simulink model "Seat_PC_Model"  (R2020a)
settings: Solver=FixedStepDiscrete  StartTime=0.0  StopTime=30  FixedStep=1  RelTol=1e-3
undefined symbols (not defined in the file or in its folder): Seat_PC_System
libraries: simulink x2
settings Model: Creator=A  LastModifiedBy=A

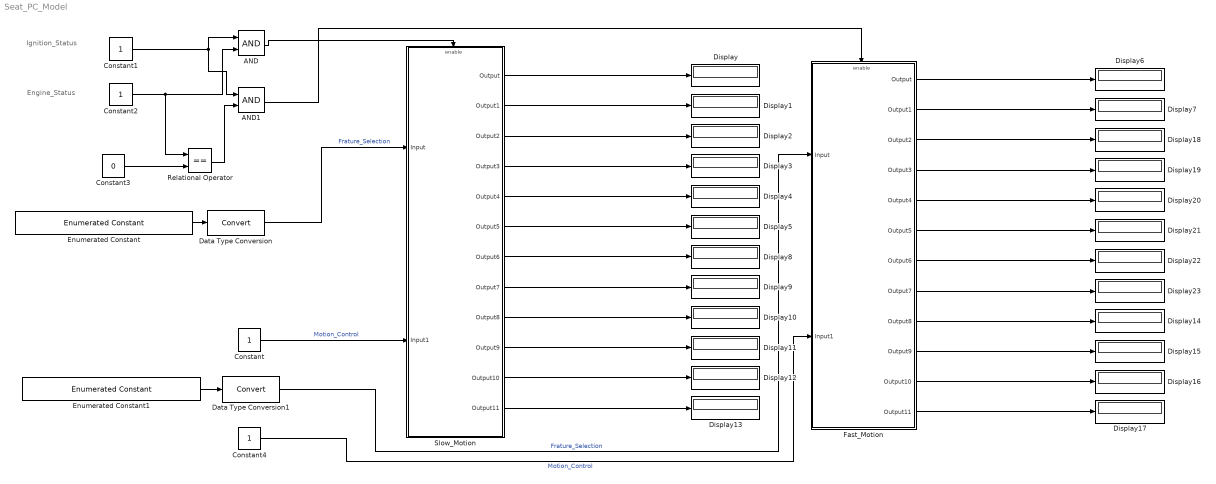
== system Seat_PC_Model ==
  note: Engine_Status
  note: Ignition_Status
  AND : Logic  AllPortsSameDT=off  OutDataTypeStr=boolean
  AND1 : Logic  AllPortsSameDT=off  OutDataTypeStr=boolean
  Constant{,1..2,4} (4 alike) : Constant  OutDataTypeStr=boolean
  Constant3 : Constant  Value=0  OutDataTypeStr=boolean
  Data Type Conversion : DataTypeConversion
  Data Type Conversion1 : DataTypeConversion
  Display{,1..23} (24 alike) : Display
  Enumerated Constant : simulink/Sources/Enumerated Constant  OutDataTypeStr=Enum:Seat_PC_System  Value=Seat_PC_System.SeatBack_FrontTilt_RearTilt_Recline_M  SampleTime=inf
  Enumerated Constant1 : simulink/Sources/Enumerated Constant  OutDataTypeStr=Enum:Seat_PC_System  Value=Seat_PC_System.Headrest_Upward_Downward_M  SampleTime=inf
  Fast_Motion : Subsystem
  Relational Operator : RelationalOperator  Operator===  OutDataTypeStr=boolean  RndMeth=Simplest
  Slow_Motion : Subsystem
  wires:
  AND/1 -> Slow_Motion/Enable
  AND1/1 -> Fast_Motion/Enable
  Constant1/1 -> AND1/1, AND/1
  Constant2/1 -> Relational Operator/1, AND/2
  Constant3/1 -> Relational Operator/2
  Relational Operator/1 -> AND1/2
  Slow_Motion/1(Output) -> Display/1
  Slow_Motion/2(Output1) -> Display1/1
  Slow_Motion/3(Output2) -> Display2/1
  Slow_Motion/4(Output3) -> Display3/1
  Slow_Motion/5(Output4) -> Display4/1
  Slow_Motion/6(Output5) -> Display5/1
  Slow_Motion/7(Output6) -> Display8/1
  Slow_Motion/8(Output7) -> Display9/1
  Slow_Motion/9(Output8) -> Display10/1
  Slow_Motion/10(Output9) -> Display11/1
  Slow_Motion/11(Output10) -> Display12/1
  Slow_Motion/12(Output11) -> Display13/1
  Fast_Motion/7(Output6) -> Display22/1
  Fast_Motion/8(Output7) -> Display23/1
  Fast_Motion/6(Output5) -> Display21/1
  Fast_Motion/12(Output11) -> Display17/1
  Fast_Motion/10(Output9) -> Display15/1
  Fast_Motion/4(Output3) -> Display19/1
  Fast_Motion/5(Output4) -> Display20/1
  Fast_Motion/11(Output10) -> Display16/1
  Fast_Motion/3(Output2) -> Display18/1
  Fast_Motion/2(Output1) -> Display7/1
  Fast_Motion/9(Output8) -> Display14/1
  Fast_Motion/1(Output) -> Display6/1
  Enumerated Constant/1 -> Data Type Conversion/1
  Data Type Conversion/1 -> Slow_Motion/1(Input)  "Frature_Selection"
  Constant/1 -> Slow_Motion/2(Input1)  "Motion_Control"
  Enumerated Constant1/1 -> Data Type Conversion1/1
  Data Type Conversion1/1 -> Fast_Motion/1(Input)  "Frature_Selection"
  Constant4/1 -> Fast_Motion/2(Input1)  "Motion_Control"

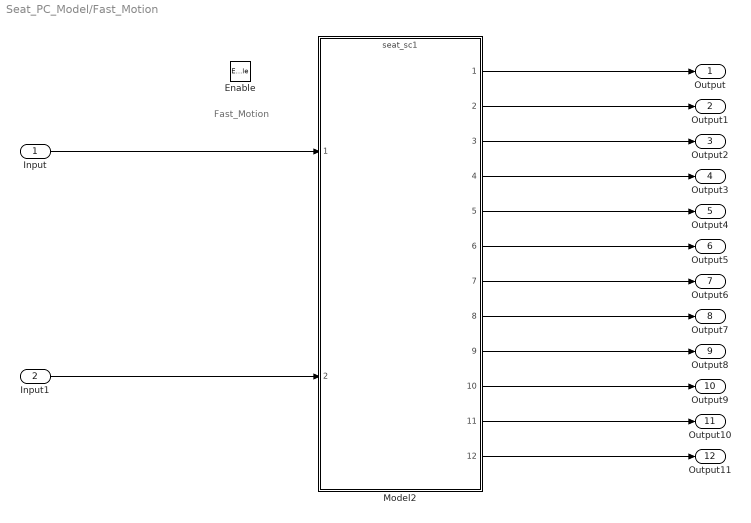
== system Seat_PC_Model/Fast_Motion ==
  note: Fast_Motion
  Input : Inport
  Input1 : Inport  Port=2
  Enable : EnablePort
  Model2 : ModelReference  ModelNameDialog=seat_sc1.slx  SimulationMode=Normal  ModelReferenceVersion=1.17
  Output : Outport
  Output1 : Outport  Port=2
  Output2 : Outport  Port=3
  Output3 : Outport  Port=4
  Output4 : Outport  Port=5
  Output5 : Outport  Port=6
  Output6 : Outport  Port=7
  Output7 : Outport  Port=8
  Output8 : Outport  Port=9
  Output9 : Outport  Port=10
  Output10 : Outport  Port=11
  Output11 : Outport  Port=12
  wires:
  Model2/1 -> Output/1
  Model2/2 -> Output1/1
  Model2/3 -> Output2/1
  Model2/4 -> Output3/1
  Model2/5 -> Output4/1
  Model2/7 -> Output6/1
  Model2/6 -> Output5/1
  Model2/8 -> Output7/1
  Model2/9 -> Output8/1
  Model2/10 -> Output9/1
  Model2/11 -> Output10/1
  Model2/12 -> Output11/1
  Input/1 -> Model2/1
  Input1/1 -> Model2/2

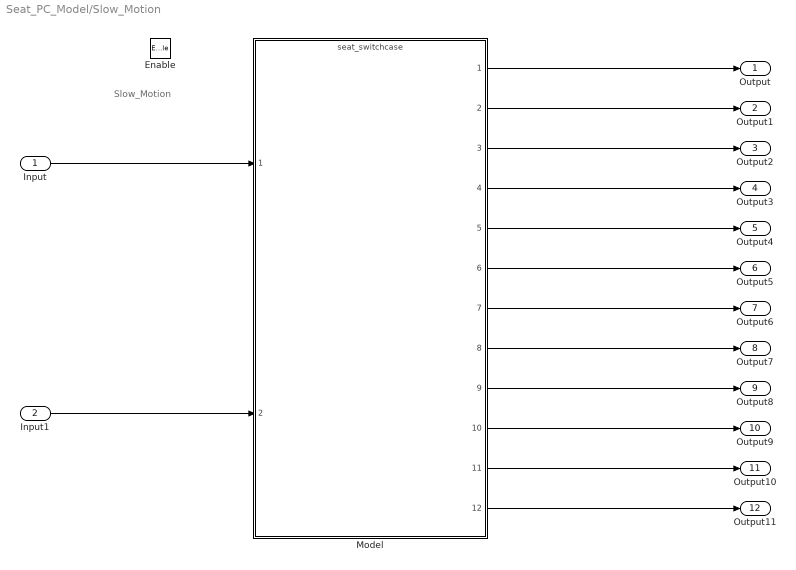
== system Seat_PC_Model/Slow_Motion ==
  note: Slow_Motion
  Input : Inport
  Input1 : Inport  Port=2
  Enable : EnablePort
  Model : ModelReference  ModelNameDialog=seat_switchcase.slx  SimulationMode=Normal  ModelReferenceVersion=1.27
  Output : Outport
  Output1 : Outport  Port=2
  Output2 : Outport  Port=3
  Output3 : Outport  Port=4
  Output4 : Outport  Port=5
  Output5 : Outport  Port=6
  Output6 : Outport  Port=7
  Output7 : Outport  Port=8
  Output8 : Outport  Port=9
  Output9 : Outport  Port=10
  Output10 : Outport  Port=11
  Output11 : Outport  Port=12
  wires:
  Model/2 -> Output1/1
  Model/1 -> Output/1
  Model/3 -> Output2/1
  Model/4 -> Output3/1
  Model/5 -> Output4/1
  Model/6 -> Output5/1
  Model/7 -> Output6/1
  Model/8 -> Output7/1
  Model/9 -> Output8/1
  Model/10 -> Output9/1
  Model/11 -> Output10/1
  Model/12 -> Output11/1
  Input/1 -> Model/1
  Input1/1 -> Model/2
